simulink model "Multi_Quad"  (R2025b)
settings: Solver=ode4  StartTime=0.0  StopTime=80.0  FixedStep=0.001  RelTol=1e-3
values from neighbouring files (symbols this model uses):
  a_hat0 = zeros(3, 4)    [init_multi.m]
  alpha = 0.5    [init_multi.m]
  D = zeros(num_agents, num_agents)    [init_multi.m]
  d0 = zeros(num_agents, 1)    [init_multi.m]
  delta = zeros(3, 4)    [init_multi.m]
  eta = 20    [init_multi.m]
  g = 9.81    [init_multi.m]
  J = diag([0.04856, 0.04856, 0.08801])    [init_multi.m]
  k_att = 0.5    [init_multi.m]
  k_d = 5    [init_multi.m]
  k_e = 5    [init_multi.m]
  k_rho = 12    [init_multi.m]
  ka = 5    [init_multi.m]
  kp = 5    [init_multi.m]
  kq = 8    [init_multi.m]
  kv = 15    [init_multi.m]
  kw = 4    [init_multi.m]
  m = 1    [init_multi.m]
  n_goal = 2    [init_multi.m]
  obs_center = [ 20,  30,  10 ... (first row only)    [init_multi.m]
  obs_rho0 = [15, 15, 15]    [init_multi.m]
  q_goal = [50; 50; 50]    [init_multi.m]
  rho0 = zeros(3, 4)    [init_multi.m]
  xInitial = [ [p0_leader; v0_leader; Q0_leader; w0_leader],               [p0_all; v0_all; Q0_all; w0_all] ]    [init_multi.m]
settings Model: Creator=ZhuanZ（无密码）  LastModifiedBy=ZhuanZ（无密码）
settings DataIOCC: ReturnWorkspaceOutputs=off

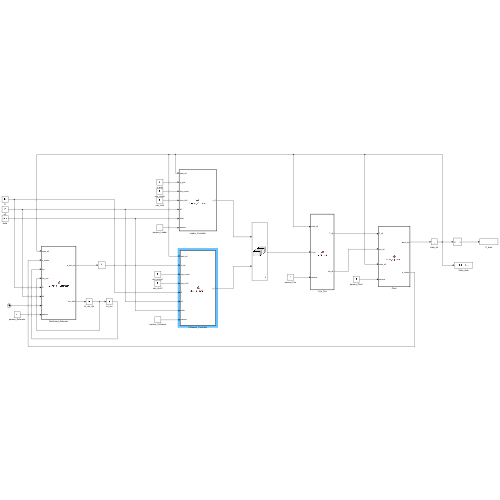
[thumbnail: Simulink's stored preview of the top-level diagram]
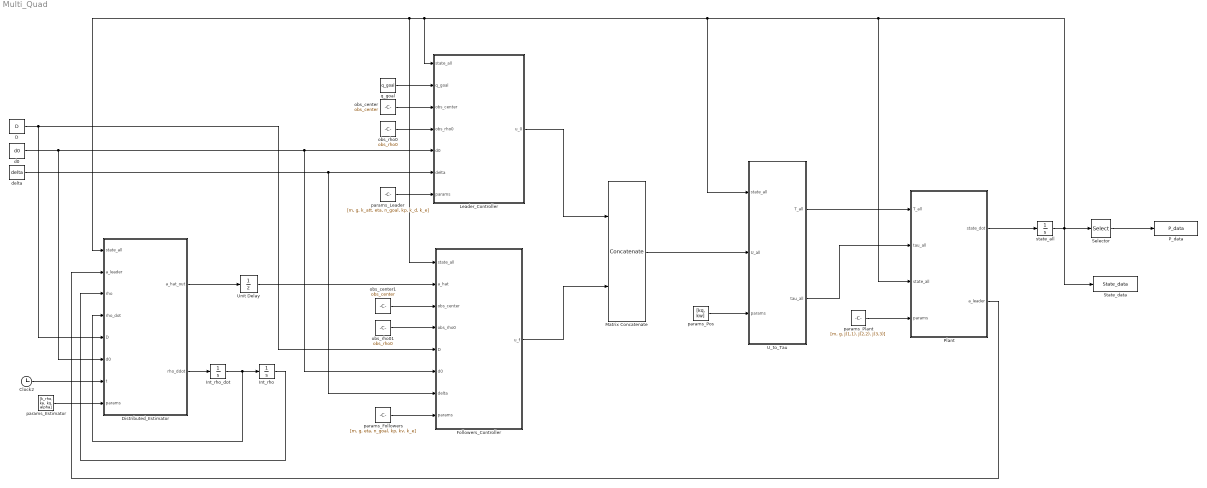
== system Multi_Quad ==
  Clock2 : Clock
  D : Constant  Value=D
  Distributed_Estimator : MATLAB Function  TreatAsAtomicUnit=on
  Followers_Controller : MATLAB Function  TreatAsAtomicUnit=on
  Int_rho : Integrator  InitialCondition=rho0
  Int_rho_dot : Integrator  InitialCondition=zeros(3, 4)
  Leader_Controller : MATLAB Function  TreatAsAtomicUnit=on
  Matrix Concatenate : Concatenate  Mode=Multidimensional array  ConcatenateDimension=2
  P_data : ToWorkspace  VariableName=P_data  SampleTime=-1
  Plant : MATLAB Function  TreatAsAtomicUnit=on
  Selector : Selector  NumberOfDimensions=2  InputPortWidth=3  IndexOptions=Index vector (dialog),Select all  Indices=1:3,1  OutputSizes=1,1
  State_data : ToWorkspace  VariableName=State_data  SampleTime=-1
  U_to_Tau : MATLAB Function  TreatAsAtomicUnit=on
  Unit Delay : UnitDelay  InitialCondition=a_hat0  SampleTime=-1  HasFrameUpgradeWarning=on
  d0 : Constant  Value=d0
  delta : Constant  Value=delta
  obs_center : Constant  Value=obs_center
  obs_center1 : Constant  Value=obs_center
  obs_rho0 : Constant  Value=obs_rho0
  obs_rho01 : Constant  Value=obs_rho0
  params_Estimator : Constant  Value=[k_rho, ka, kq, alpha]
  params_Followers : Constant  Value=[m, g, eta, n_goal, kp, kv, k_e]
  params_Leader : Constant  Value=[m, g, k_att, eta, n_goal, kp, k_d, k_e]
  params_Plant : Constant  Value=[m, g, J(1,1), J(2,2), J(3,3)]
  params_Pos : Constant  Value=[kq, kw]
  q_goal : Constant  Value=q_goal
  state_all : Integrator  InitialCondition=xInitial
  wires:
  params_Leader/1 -> Leader_Controller/7(params)
  obs_rho0/1 -> Leader_Controller/4(obs_rho0)
  obs_center/1 -> Leader_Controller/3(obs_center)
  q_goal/1 -> Leader_Controller/2(q_goal)
  params_Followers/1 -> Followers_Controller/8(params)
  delta/1 -> Followers_Controller/7(delta), Leader_Controller/6(delta)
  d0/1 -> Leader_Controller/5(d0), Followers_Controller/6(d0), Distributed_Estimator/6(d0)
  D/1 -> Followers_Controller/5(D), Distributed_Estimator/5(D)
  obs_rho01/1 -> Followers_Controller/4(obs_rho0)
  obs_center1/1 -> Followers_Controller/3(obs_center)
  Distributed_Estimator/2(rho_ddot) -> Int_rho_dot/1
  Int_rho_dot/1 -> Int_rho/1, Distributed_Estimator/4(rho_dot)
  Int_rho/1 -> Distributed_Estimator/3(rho)
  Clock2/1 -> Distributed_Estimator/7(t)
  params_Estimator/1 -> Distributed_Estimator/8(params)
  Leader_Controller/1(u_0) -> Matrix Concatenate/1
  Followers_Controller/1(u_f) -> Matrix Concatenate/2
  Matrix Concatenate/1 -> U_to_Tau/2(U_all)
  params_Pos/1 -> U_to_Tau/3(params)
  U_to_Tau/1(T_all) -> Plant/1(T_all)
  U_to_Tau/2(tau_all) -> Plant/2(tau_all)
  params_Plant/1 -> Plant/4(params)
  Plant/1(state_dot) -> state_all/1
  state_all/1 -> State_data/1, Selector/1, U_to_Tau/1(state_all), Leader_Controller/1(state_all), Distributed_Estimator/1(state_all), Followers_Controller/1(state_all), Plant/3(state_all)
  Plant/2(a_leader) -> Distributed_Estimator/2(a_leader)
  Selector/1 -> P_data/1
  Distributed_Estimator/1(a_hat_out) -> Unit Delay/1
  Unit Delay/1 -> Followers_Controller/2(a_hat)

== matlab function Multi_Quad/Leader_Controller ==
  data: state_all input; u_0 output; q_goal input; obs_center input; obs_rho0 input; d0 input; delta input; params input
function u_0 = Leader_Controller(state_all, q_goal, obs_center, obs_rho0, d0, delta, params)
    % =====================================================================
    % 输入说明：
    % state_all:   13 x (N+1) 矩阵，全状态矩阵。第 1 列为领航者x_followers: 13xN 矩阵，所有跟随者的完整状态 (每一列是一架跟随者)
    % q_goal:      3x1 向量，全局目标点坐标
    % obs_center:  3x1 向量，障碍物中心坐标
    % obs_rho0:    标量，障碍物警戒半径
    % d0:          Nx1 向量，表示跟随者是否与领航者双向连通 (init_multi.m 中的 d0)
    % delta:       3xN 矩阵，跟随者的期望编队偏移量 (init_multi.m 中的 delta)
    % params:      1x8 数组，[m, g, k_att, eta, n_goal, kp, k_d, k_e]
    %
    % 输出说明：
    % u_0:         3x1 向量，领航者产生的外环虚拟合力 (输出给姿态解算模块)
    % =====================================================================

    % 1. 解析参数
    m       = params(1);
    g       = params(2);
    k_att   = params(3);
    eta     = params(4);
    n_goal  = params(5);
    kp      = params(6);
    k_d     = params(7);
    k_e     = params(8);   

    epsilon = 1e-6; % 防止除以 0 的微小常数

    % 2. 内部切片：提取状态
    p_0 = state_all(1:3, 1);
    v_0 = state_all(4:6, 1);
    
    p_followers = state_all(1:3, 2:end); 
    num_followers = size(p_followers, 2);

    %% 3. 重力补偿
    e3 = [0; 0; 1];
    u_g = m * g * e3;

    %% 4. 目标点引力 F_att (Pan 论文)
    rho_g = norm(p_0 - q_goal);
    n_pg = (p_0 - q_goal) / (rho_g + epsilon);
    F_att = -k_att * rho_g * n_pg; 
    
    % [新增限幅] 防止远距离起飞时引力大到让飞机翻车
    if norm(F_att) > 8
        F_att = (F_att / norm(F_att)) * 8;
    end

%% 5 & 6. 多障碍物势场叠加 (F_rep 和 F_e)
    F_rep_total = zeros(3, 1);
    F_e_total = zeros(3, 1);
    num_obs = size(obs_center, 2); % 获取障碍物数量
    
    for k = 1:num_obs
        rho_o = norm(p_0 - obs_center(:, k));
        n_op = (p_0 - obs_center(:, k)) / (rho_o + epsilon);
        
        if rho_o <= obs_rho0(k)
            % A. 斥力计算 (当前障碍物)
            term1 = eta * (1/rho_o - 1/obs_rho0(k)) * (rho_g^n_goal) / (rho_o^2);
            F_rep1 = term1 * n_op;
            term2 = (n_goal / 2) * eta * (1/rho_o - 1/obs_rho0(k))^2 * (rho_g^(n_goal-1));
            F_rep2 = term2 * (-n_pg);
            F_rep_k = F_rep1 + F_rep2;
            
            if norm(F_rep_k) > 15
                F_rep_k = (F_rep_k / norm(F_rep_k)) * 15;
            end
            F_rep_total = F_rep_total + F_rep_k; % 斥力叠加
            
            % B. 防死锁旋转力计算 (当前障碍物)
            F_e_k = zeros(3, 1);
            if norm(F_att) > epsilon && norm(F_rep_k) > epsilon
                cos_theta = dot(F_att, F_rep_k) / (norm(F_att) * norm(F_rep_k));
                smooth_factor = exp(5 * (-cos_theta - 1));
                F_e_k = k_e * smooth_factor * (obs_rho0(k) - rho_o) * cross(n_op, e3);
            end
            F_e_total = F_e_total + F_e_k; % 旋转力叠加
        end
    end

    % %% 7. 跟随者掉队的反馈拉扯力 F_feedback (Wang 论文一致性协议)
    % sum_err = zeros(3, 1);
    % for j = 1:num_followers
    %     if d0(j) == 1 % 如果 j 号机和领航者双向通信
    %         p_j = p_followers(:, j);
    %         % 计算位置误差：领航者实际领先量 vs 期望领先量 (-delta_j)
    %         err_j = p_0 - p_j + delta(:, j); 
    %         sum_err = sum_err + err_j;
    %     end
    % end
    % F_feedback = kp * tanh(sum_err);

    %% 8. 速度阻尼项 F_damp
    F_damp = -k_d * v_0;

    %% 9. 最终合成虚拟合力 (加入了 F_e)
    u_0 = u_g + F_att + F_rep_total + F_e_total + F_damp;

    % =======================================================
    % 🚨 物理推力保护锁：限制最大加速度不超过 50 m/s^2 (约 5G)
    % 彻底掐断 APF 势场距离爆炸导致的 $10^{173}$ 坐标！
    % =======================================================
    max_thrust = 50 * m; 
    if norm(u_0) > max_thrust
        u_0 = (u_0 / norm(u_0)) * max_thrust;
    end
end

== matlab function Multi_Quad/Followers_Controller ==
  data: state_all input; u_f output; a_hat input; obs_center input; obs_rho0 input; D input; d0 input; delta input; params input
function u_f = Followers_Controller(state_all, a_hat, obs_center, obs_rho0, D, d0, delta, params)
    % =====================================================================
    % 输入说明：
    % state_all:   13 x (N+1) 全状态矩阵。第1列为领航者，第2~N+1列为跟随者
    % a_hat:       3 x N 矩阵，估计器算出的领航者加速度前馈量
    % obs_center:  3x1 向量，障碍物中心坐标
    % obs_rho0:    标量，障碍物警戒半径
    % D:           N x N 跟随者之间的邻接拓扑矩阵
    % d0:          N x 1 向量，表示各跟随者是否与领航者直接连通
    % delta:       3 x N 矩阵，期望编队偏移量
    % params:      1 x 7 数组，[m, g, eta, n_goal, kp, kv, k_e]
    %
    % 输出说明：
    % u_f:         3 x N 矩阵，所有跟随者的虚拟合力
    % =====================================================================

    % 1. 解析参数
    m       = params(1);
    g       = params(2);
    eta     = params(3);
    n_goal  = params(4);
    kp      = params(5);
    kv      = params(6);
    k_e     = params(7);

    num_followers = size(state_all, 2) - 1;
    u_f = zeros(3, num_followers); % 初始化输出矩阵
    epsilon = 1e-6; 

    % 2. 提取状态
    p_0 = state_all(1:3, 1);
    v_0 = state_all(4:6, 1);
    
    p_f = state_all(1:3, 2:end); 
    v_f = state_all(4:6, 2:end);

    % 先算出所有跟随者的绝对误差 (相对领航者的理想位置)
    % err_p_i = p_i - p_0 - delta_i
    err_p = zeros(3, num_followers);
    err_v = zeros(3, num_followers);
    for i = 1:num_followers
        err_p(:, i) = p_f(:, i) - p_0 - delta(:, i);
        err_v(:, i) = v_f(:, i) - v_0; % 期望速度相对领航者为 0
    end

    %% 核心：遍历计算每一个跟随者的受力
    e3 = [0; 0; 1];
    
    for i = 1:num_followers
        
        % -----------------------------------------------------------------
        % A. 计算 Wang 的一致性协议控制力 (F_cons)
        % -----------------------------------------------------------------
        sum_p = zeros(3, 1);
        sum_v = zeros(3, 1);
        
        % A.1 来自领航者的误差拉力 (如果 d0=1)
        sum_p = sum_p + d0(i) * err_p(:, i);
        sum_v = sum_v + d0(i) * err_v(:, i);
        
        % A.2 来自邻居跟随者的误差拉力
        for j = 1:num_followers
            if D(i, j) == 1
                % (p_i^e - p_j^e) 等价于算两机的相对位置与期望相对位置的差
                sum_p = sum_p + D(i, j) * (err_p(:, i) - err_p(:, j));
                sum_v = sum_v + D(i, j) * (err_v(:, i) - err_v(:, j));
            end
        end
        
        % 带限幅的一致性内部弹簧力 (包含了位置与速度阻尼)
        F_cons = -kp * tanh(sum_p) - kv * tanh(sum_v);

        % -----------------------------------------------------------------
        % B & C. 多障碍物势场叠加 (F_rep 和 F_e)
        % -----------------------------------------------------------------
        F_rep_total = zeros(3, 1);
        F_e_total = zeros(3, 1);
        in_alert_zone = false; % 标记是否进入了任何障碍物的警戒圈
        num_obs = size(obs_center, 2);
        
        for k = 1:num_obs
            rho_o = norm(p_f(:, i) - obs_center(:, k));
            n_op = (p_f(:, i) - obs_center(:, k)) / (rho_o + epsilon); 
            
            if rho_o <= obs_rho0(k)
                in_alert_zone = true; % 只要进入任何一个，就触发避震标志
                
                % 斥力叠加
                term1 = (eta * 1000) * (1/rho_o - 1/obs_rho0(k)) / (rho_o^2);
                F_rep_k = term1 * n_op;
                if norm(F_rep_k) > 20
                    F_rep_k = (F_rep_k / norm(F_rep_k)) * 20;
                end
                F_rep_total = F_rep_total + F_rep_k;
                
                % 旋转防死锁力叠加
                F_e_k = zeros(3, 1);
                if norm(F_cons) > epsilon && norm(F_rep_k) > epsilon
                    cos_theta = dot(F_cons, F_rep_k) / (norm(F_cons) * norm(F_rep_k));
                    smooth_factor = exp(5 * (-cos_theta - 1));
                    F_e_k = k_e * smooth_factor * (obs_rho0(k) - rho_o) * cross(n_op, e3);
                end
                F_e_total = F_e_total + F_e_k;
            end
        end

        % -----------------------------------------------------------------
        % D. 最终合力组装
        % -----------------------------------------------------------------
        a_hat_safe = max(min(a_hat(:, i), 8), -8); 
        
        % 统一避震器：无论受几个障碍物影响，仅施加一次阻尼吸收震荡
        F_obs_damp = zeros(3, 1);
        if in_alert_zone
            F_obs_damp = -3 * err_v(:, i); 
        end
        
        u_f(:, i) = m * (g * e3 + a_hat_safe) + F_cons + F_rep_total + F_e_total + F_obs_damp;
        
        % 物理推力保护锁
        max_thrust = 50 * m; 
        if norm(u_f(:, i)) > max_thrust
            u_f(:, i) = (u_f(:, i) / norm(u_f(:, i))) * max_thrust;
        end
    end
end

== matlab function Multi_Quad/Distributed_Estimator ==
  data: state_all input; a_hat_out output; a_leader input; rho input; rho_dot input; D input; d0 input; t input; params input; rho_ddot output
function [a_hat_out, rho_ddot] = Distributed_Estimator(state_all, a_leader, rho, rho_dot, D, d0, t, params)
    
    % =====================================================================
    % 输入说明：
    % state_all: 13 x (N+1) 全状态矩阵。第 1 列为领航者
    % a_leader:  3 x 1 领航者的实际加速度 (从 Plant 模块直接接过来)
    % rho:       3 x N 估计器内部状态 (来自外接的积分器)
    % rho_dot:   3 x N 估计器状态的一阶导数 (来自外接的积分器)
    % D:         N x N 跟随者邻接矩阵
    % d0:        N x 1 领航者连接权重向量
    % t:         1 x 1 仿真时钟 (Clock 模块输入)
    % params:    1 x 4 估计器增益数组 [k_rho, k_a, k_q, alpha]
    %
    % 输出说明：
    % a_hat_out: 3 x N 计算出的领航者加速度前馈量 (输出给 Follower_Controller)
    % rho_ddot:  3 x N 状态的二阶导数 (输出给两个串联的积分器)
    % =====================================================================

    % 1. 解析增益参数
    k_rho = params(1);
    k_a   = params(2);
    k_q   = params(3);
    alpha = params(4);
    
    num_followers = size(rho, 2);
    
    % 领航者状态解构
    p_0 = state_all(1:3, 1);
    v_0 = state_all(4:6, 1);
    a_leader = max(min(a_leader, 8), -8);
    jerk_0 = zeros(3, 1); 
    
    % =====================================================================
    % 🚨 安全补丁 1：给时变衰减函数加“底板”
    % 防止 t 变大时 eps_t 趋于 0，导致除法将微小噪声放大到无穷大！
    % =====================================================================
    eps_t = exp(-alpha * t) + 0.5; 
    
    a_hat_out = zeros(3, num_followers);
    a_hat_dot = zeros(3, num_followers);
    rho_ddot  = zeros(3, num_followers);
    
    for i = 1:num_followers
        a_hat_out(:, i) = k_rho * tanh(rho(:, i));
        a_hat_dot(:, i) = k_rho * (1 - tanh(rho(:, i)).^2) .* rho_dot(:, i);
    end
    
    for i = 1:num_followers
        sum_a = zeros(3, 1);
        sum_a_dot = zeros(3, 1);
        
        for j = 1:num_followers
            if D(i, j) == 1
                sum_a     = sum_a     + D(i, j) * (a_hat_out(:, i) - a_hat_out(:, j));
                sum_a_dot = sum_a_dot + D(i, j) * (a_hat_dot(:, i) - a_hat_dot(:, j));
            end
        end
        
        term_leader_a     = d0(i) * (a_hat_out(:, i) - a_leader);
        term_leader_a_dot = d0(i) * (a_hat_dot(:, i) - jerk_0);
        
        term_sum_1 = sum_a + term_leader_a;             
        term_sum_2 = sum_a_dot + term_leader_a_dot;     
        
        Xi_i = tanh(rho(:, i)) .* rho_dot(:, i);
        
        % 平滑奇异点保护 (安全底线 0.05)
        Upsilon_i = k_rho * (1 - tanh(rho(:, i)).^2) + 0.05; 
        inv_Upsilon = 1 ./ Upsilon_i;
        
        part1 = (2 * Xi_i - 1) .* rho_dot(:, i);
        
        bracket = (k_q / k_rho) * (term_sum_1 + term_sum_2) + ...
                  (k_a / k_rho) * tanh(term_sum_1 / eps_t) + ...
                  (term_sum_2 / eps_t);
                  
        % 计算原始的 rho_ddot
        rho_ddot_raw = part1 - inv_Upsilon .* bracket;
        
        % =================================================================
        % 🚨 安全补丁 2：恢复你原代码中的“终极硬限幅”
        % 保护数值解算器，防止瞬态尖峰撕裂系统步长
        % =================================================================
        rho_ddot(:, i) = max(min(rho_ddot_raw, 2000), -2000); 
    end
end

== matlab function Multi_Quad/U_to_Tau ==
  data: state_all input; T_all output; U_all input; params input; tau_all output
function [T_all, tau_all] = U_to_Tau(state_all, U_all, params)
    % =====================================================================
    % 输入说明：
    % state_all: 13 x (N+1) 全状态矩阵。第 1 列为领航者，后续为跟随者
    % U_all:     3 x (N+1) 所有无人机的虚拟合力矩阵 (通过 Matrix Concatenate 合并)
    % params:    1 x 2 数组，姿态环控制增益 [k_t, k_w] (对应 init 中的 [kq, kw])
    %
    % 输出说明：
    % T_all:     1 x (N+1) 标量数组，所有无人机的总推力大小
    % tau_all:   3 x (N+1) 矩阵，所有无人机的三轴控制力矩
    % =====================================================================

    % 1. 解析姿态环增益
    k_t = params(1);
    k_w = params(2);
    
    num_agents = size(state_all, 2); % 包含了 Leader 和 所有 Followers
    
    % 初始化输出
    T_all   = zeros(1, num_agents);
    tau_all = zeros(3, num_agents);
    
    for i = 1:num_agents
        u_c    = U_all(:, i);
        Q_curr = state_all(7:10, i);  % 当前四元数姿态 [q0; q1; q2; q3]
        w_curr = state_all(11:13, i); % 当前角速度
        
        %% --- 步骤 1: 计算推力大小 T ---
        q0 = Q_curr(1); q1 = Q_curr(2); q2 = Q_curr(3); q3 = Q_curr(4);
        R_e3 = [ 2 * (q1*q3 + q0*q2);
                 2 * (q2*q3 - q0*q1);
                 q0^2 - q1^2 - q2^2 + q3^2 ];
                 
        % 🚨 真正的工业级推力映射：将期望推力投影到当前的实际姿态Z轴上！
        % 这样就算姿态没跟上，垂直方向的升力也绝对不会超过期望值，彻底消除 Ballooning！
        T_all(i) = dot(u_c, R_e3);
        
        % 物理底线保护
        if T_all(i) < 1.0
            T_all(i) = 1.0; 
        end
        
        % 依然需要计算 norm_uc 用于下面步骤 2 的归一化
        norm_uc = norm(u_c);
        if norm_uc < 1e-6
            norm_uc = 1e-6; 
        end
        
        %% --- 步骤 2: 计算指令姿态 Qc ---
        u_z = u_c(3);
        % 🚨 鲁棒的推力矢量转四元数算法 (完美避免 sigma_c 趋于 0 的奇异点)
        q_raw = [norm_uc + u_z; -u_c(2); u_c(1); 0];
        Qc = q_raw / norm(q_raw);
        
        %% --- 步骤 3: 计算姿态误差 Qe = Qc^{-1} \otimes Q_curr ---
        % Qc 的逆即为其共轭 (假设 Qc 已归一化): Qc^{-1} = [Qc(1); -Qc(2:4)]
        Qc_inv = [Qc(1); -Qc(2:4)];
        
        p0 = Qc_inv(1); pv = Qc_inv(2:4);
        r0 = Q_curr(1); rv = Q_curr(2:4);
        
        % 四元数乘法解算，实际上我们只需要误差四元数的虚部向量 (Qe_vec) 
        % 来参与 PD 控制，实部 Qe_0 通常用于判断旋转方向，这里可省略
        Qe_vec = p0 * rv + r0 * pv + cross(pv, rv);
        
        %% --- 步骤 4: 计算简化的控制力矩 tau ---
        % 抛弃高频噪声前馈与陀螺仪补偿，使用最鲁棒的纯 PD 闭环
        tau_all(:, i) = -k_t * Qe_vec - k_w * w_curr;
    end
end

== matlab function Multi_Quad/Plant ==
  data: T_all input; state_dot output; tau_all input; state_all input; params input; a_leader output
function [state_dot, a_leader] = Plant_Dynamics(T_all, tau_all, state_all, params)
    % =====================================================================
    % 输入说明：
    % T_all:     1 x (N+1) 标量数组，所有无人机的总推力
    % tau_all:   3 x (N+1) 矩阵，所有无人机的三轴控制力矩
    % state_all: 13 x (N+1) 全状态矩阵。第 1 列为领航者
    % params:    1 x 5 物理参数数组 [m, g, Jx, Jy, Jz]
    %
    % 输出说明：
    % state_dot: 13 x (N+1) 状态导数矩阵 (输出给纯积分器 Integrator)
    % a_leader:  3 x 1 领航者的实际加速度 (输出给 Estimator 模块)
    % =====================================================================

    % 1. 解析物理参数
    m = params(1);
    g = params(2);
    % 还原惯性张量矩阵 J (对角阵)
    J = diag([params(3), params(4), params(5)]);

    num_agents = size(state_all, 2);
    
    % 初始化输出
    state_dot = zeros(13, num_agents);
    a_leader  = zeros(3, 1);

    % 遍历每一架无人机计算物理引擎
    for i = 1:num_agents
        
        % 提取当前状态
        p = state_all(1:3, i);
        v = state_all(4:6, i);
        Q = state_all(7:10, i); % 四元数 [q0, q1, q2, q3]^T
        w = state_all(11:13, i);

        % 🚨 极其重要：强制归一化四元数！
        % 防止 Simulink 数值积分漂移导致物理引擎推力无限放大！
        Q = Q / norm(Q);
        
        T = T_all(i);
        tau = tau_all(:, i);

        %% --- 步骤 1: 旋转矩阵与平动动力学 (牛顿定律) ---
        q0 = Q(1); q1 = Q(2); q2 = Q(3); q3 = Q(4);
        
        % 计算机身 Z 轴在全局坐标系下的朝向 (即旋转矩阵 R 的第三列 R*e3)
        R_e3 = [ 2 * (q1*q3 + q0*q2);
                 2 * (q2*q3 - q0*q1);
                 q0^2 - q1^2 - q2^2 + q3^2 ];
             
        % 计算加速度 v_dot
        % m * v_dot = -m * g * e3 + T * (R * e3)
        v_dot = -g * [0; 0; 1] + (T / m) * R_e3;
        
        %% --- 步骤 2: 平动运动学 ---
        p_dot = v;
        
        %% --- 步骤 3: 转动运动学 (四元数微分方程) ---
        wx = w(1); wy = w(2); wz = w(3);
        % Q_dot = 1/2 * Q \otimes [0; w] 写成矩阵相乘形式：
        Q_dot = 0.5 * [ -q1, -q2, -q3;
                         q0, -q3,  q2;
                         q3,  q0, -q1;
                        -q2,  q1,  q0 ] * [wx; wy; wz];

        %% --- 步骤 4: 转动动力学 (欧拉方程) ---
        % J * w_dot = -cross(w, J*w) + tau
        w_dot = J \ (tau - cross(w, J * w));
        
        %% --- 步骤 5: 组装当前飞机的状态导数 ---
        state_dot(:, i) = [p_dot; v_dot; Q_dot; w_dot];
        
        %% --- 步骤 6: 专门提取领航者的加速度给 Estimator ---
        if i == 1
            a_leader = v_dot;
        end
    end
end
